simulink model "Ex_3"  (R2023b)
settings: Solver=VariableStepAuto  StartTime=0.0  StopTime=10.0  RelTol=1e-3
undefined symbols (not defined in the file): X, Y, Z
libraries: nesl_utility x21, sm_lib x20, robotcorelib x2, simulink x2
settings Model: Creator=aless  LastModifiedBy=aless

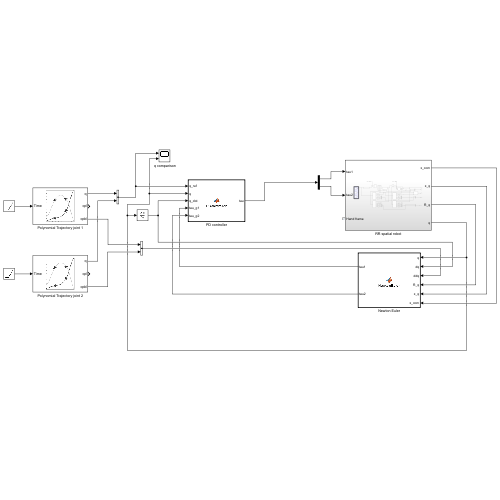
[thumbnail: Simulink's stored preview of the top-level diagram]
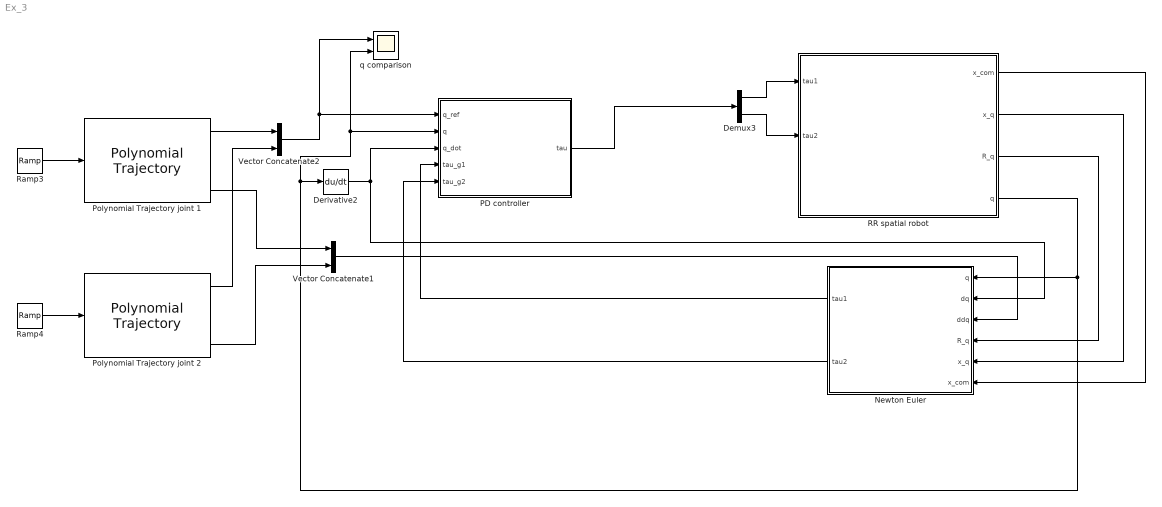
== system Ex_3 ==
  " q comparison" : Scope  NumInputPorts=2
  Demux3 : Demux  Outputs=2
  Derivative2 : Derivative
  Newton Euler : MATLAB Function  TreatAsAtomicUnit=on
  PD controller : MATLAB Function  TreatAsAtomicUnit=on
  Polynomial Trajectory joint 1 : robotcorelib/Polynomial Trajectory  WaypointSource=Internal  Waypoints=[ deg2rad(-25), deg2rad(100)]  TimePoints=[ 0, 10]  TimeInterval=[ 1, 4 ]  Method=Cubic Polynomial  ParameterSource=Internal  VelocityBoundaryCondition=zeros( 1, 2 )  AccelerationBoundaryCondition=zeros( 2, 5 )  SimulateUsing=Interpreted execution
  Polynomial Trajectory joint 2 : robotcorelib/Polynomial Trajectory  WaypointSource=Internal  Waypoints=[ deg2rad(45), deg2rad(80)]  TimePoints=[ 0, 10]  TimeInterval=[ 1, 4 ]  Method=Cubic Polynomial  ParameterSource=Internal  VelocityBoundaryCondition=zeros( 1, 2 )  AccelerationBoundaryCondition=zeros( 2, 5 )  SimulateUsing=Interpreted execution
  RR spatial robot : Subsystem
  Ramp3 : simulink/Sources/Ramp  slope=1  start=0  InitialOutput=0
  Ramp4 : simulink/Sources/Ramp  slope=1  start=0  InitialOutput=0
  Vector Concatenate1 : Concatenate
  Vector Concatenate2 : Concatenate
  wires:
  Demux3/2 -> RR spatial robot/2(tau2)
  Polynomial Trajectory joint 1/1 -> Vector Concatenate2/1
  Polynomial Trajectory joint 2/1 -> Vector Concatenate2/2
  Vector Concatenate1/1 -> Newton Euler/3(ddq)
  Polynomial Trajectory joint 1/3 -> Vector Concatenate1/1
  Newton Euler/2(tau2) -> PD controller/5(tau_g2)
  PD controller/1(tau) -> Demux3/1
  Polynomial Trajectory joint 2/3 -> Vector Concatenate1/2
  RR spatial robot/3(R_q) -> Newton Euler/4(R_q)
  Newton Euler/1(tau1) -> PD controller/4(tau_g1)
  RR spatial robot/4(q) -> Derivative2/1, " q comparison"/2, PD controller/2(q), Newton Euler/1(q)
  Ramp4/1 -> Polynomial Trajectory joint 2/1
  Ramp3/1 -> Polynomial Trajectory joint 1/1
  Derivative2/1 -> Newton Euler/2(dq), PD controller/3(q_dot)
  Demux3/1 -> RR spatial robot/1(tau1)
  Vector Concatenate2/1 -> " q comparison"/1, PD controller/1(q_ref)
  RR spatial robot/1(x_com) -> Newton Euler/6(x_com)
  RR spatial robot/2(x_q) -> Newton Euler/5(x_q)

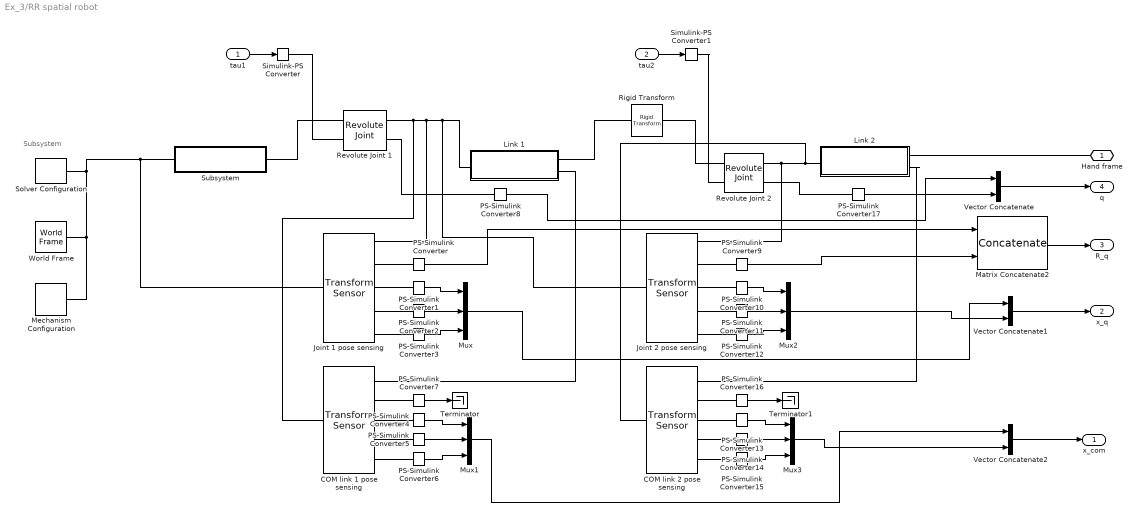
== system Ex_3/RR spatial robot ==
  note: Subsystem
  tau1 : Inport
  tau2 : Inport  Port=2
  COM link 1 pose sensing : sm_lib/Frames and Transforms/Transform Sensor  MeasurementFrame=Base  RotationSequence=XYX  SenseAngle=off  SenseAxis=off  SenseQ=off  SenseR=on  SenseRotationSequence=off  SenseOmegaX=off  SenseOmegaY=off  SenseOmegaZ=off  SenseOmega=off  SenseQDot=off  SenseRDot=off  SenseRotationSequenceDot=off  SenseAlphaX=off  SenseAlphaY=off  SenseAlphaZ=off  SenseAlpha=off  SenseQDDot=off  SenseRDDot=off  SenseX=on  SenseY=on  SenseZ=on  SenseXYZ=off  SenseRad=off  SenseAzim=off  SenseDist=off  SenseInc=off  SenseXDot=off  SenseYDot=off  SenseZDot=off  SenseXYZDot=off  SenseRadDot=off  SenseAzimDot=off  SenseDistDot=off  SenseIncDot=off  SenseXDDot=off  SenseYDDot=off  SenseZDDot=off  SenseXYZDDot=off  SenseRadDDot=off  SenseAzimDDot=off  SenseDistDDot=off  SenseIncDDot=off
  COM link 2 pose sensing : sm_lib/Frames and Transforms/Transform Sensor  MeasurementFrame=Base  RotationSequence=XYX  SenseAngle=off  SenseAxis=off  SenseQ=off  SenseR=on  SenseRotationSequence=off  SenseOmegaX=off  SenseOmegaY=off  SenseOmegaZ=off  SenseOmega=off  SenseQDot=off  SenseRDot=off  SenseRotationSequenceDot=off  SenseAlphaX=off  SenseAlphaY=off  SenseAlphaZ=off  SenseAlpha=off  SenseQDDot=off  SenseRDDot=off  SenseX=on  SenseY=on  SenseZ=on  SenseXYZ=off  SenseRad=off  SenseAzim=off  SenseDist=off  SenseInc=off  SenseXDot=off  SenseYDot=off  SenseZDot=off  SenseXYZDot=off  SenseRadDot=off  SenseAzimDot=off  SenseDistDot=off  SenseIncDot=off  SenseXDDot=off  SenseYDDot=off  SenseZDDot=off  SenseXYZDDot=off  SenseRadDDot=off  SenseAzimDDot=off  SenseDistDDot=off  SenseIncDDot=off
  Joint 1 pose sensing : sm_lib/Frames and Transforms/Transform Sensor  MeasurementFrame=Base  RotationSequence=XYX  SenseAngle=off  SenseAxis=off  SenseQ=off  SenseR=on  SenseRotationSequence=off  SenseOmegaX=off  SenseOmegaY=off  SenseOmegaZ=off  SenseOmega=off  SenseQDot=off  SenseRDot=off  SenseRotationSequenceDot=off  SenseAlphaX=off  SenseAlphaY=off  SenseAlphaZ=off  SenseAlpha=off  SenseQDDot=off  SenseRDDot=off  SenseX=on  SenseY=on  SenseZ=on  SenseXYZ=off  SenseRad=off  SenseAzim=off  SenseDist=off  SenseInc=off  SenseXDot=off  SenseYDot=off  SenseZDot=off  SenseXYZDot=off  SenseRadDot=off  SenseAzimDot=off  SenseDistDot=off  SenseIncDot=off  SenseXDDot=off  SenseYDDot=off  SenseZDDot=off  SenseXYZDDot=off  SenseRadDDot=off  SenseAzimDDot=off  SenseDistDDot=off  SenseIncDDot=off
  Joint 2 pose sensing : sm_lib/Frames and Transforms/Transform Sensor  MeasurementFrame=Base  RotationSequence=XYX  SenseAngle=off  SenseAxis=off  SenseQ=off  SenseR=on  SenseRotationSequence=off  SenseOmegaX=off  SenseOmegaY=off  SenseOmegaZ=off  SenseOmega=off  SenseQDot=off  SenseRDot=off  SenseRotationSequenceDot=off  SenseAlphaX=off  SenseAlphaY=off  SenseAlphaZ=off  SenseAlpha=off  SenseQDDot=off  SenseRDDot=off  SenseX=on  SenseY=on  SenseZ=on  SenseXYZ=off  SenseRad=off  SenseAzim=off  SenseDist=off  SenseInc=off  SenseXDot=off  SenseYDot=off  SenseZDot=off  SenseXYZDot=off  SenseRadDot=off  SenseAzimDot=off  SenseDistDot=off  SenseIncDot=off  SenseXDDot=off  SenseYDDot=off  SenseZDDot=off  SenseXYZDDot=off  SenseRadDDot=off  SenseAzimDDot=off  SenseDistDDot=off  SenseIncDDot=off
  Link 1 : Subsystem
  Link 2 : Subsystem
  Matrix Concatenate2 : Concatenate  Mode=Multidimensional array  ConcatenateDimension=3
  Mechanism Configuration : sm_lib/Utilities/Mechanism Configuration  UniformGravity=Constant  GravityVector=[0 0 -9.80665]  GravityVectorUnits=m/s^2  LinearizationDelta=0.001  JointModeTransitionNonlinearIterations=2
  Mux{,1..3} (4 alike) : Mux  Inputs=3
  PS-Simulink Converter{,1..17} (18 alike) : nesl_utility/PS-Simulink Converter  PhysicalDomain=network_engine_domain  SubClassName=ps_output  LeftPortType=input  RightPortType=output  PseudoPeriodic=off  Frequencies=[]  VectorFormat=inherit  Unit=inherit  AffineConversion=off
  Revolute Joint 1 : sm_lib/Joints/Revolute Joint  JointMode=Normal  SenseConstraintForce=off  SenseConstraintForceX=off  SenseConstraintForceY=off  SenseConstraintForceZ=off  SenseConstraintTorque=off  SenseConstraintTorqueX=off  SenseConstraintTorqueY=off  SenseConstraintTorqueZ=off  SenseTotalForce=off  SenseTotalForceX=off  SenseTotalForceY=off  SenseTotalForceZ=off  SenseTotalTorque=off  SenseTotalTorqueX=off  SenseTotalTorqueY=off  SenseTotalTorqueZ=off  CompositeWrenchDir=FollowerOnBase  CompositeWrenchFrame=BaseFrame  EquilibriumPosition=0  EquilibriumPositionUnits=deg  SpringStiffness=0  SpringStiffnessUnits=N*m/deg  DampingCoefficient=0  DampingCoefficientUnits=N*m*s/rad  TorqueActuationMode=InputTorque  MotionActuationMode=ComputedMotion  SensePosition=on  SenseVelocity=off  SenseAcceleration=off  SenseTorqueForce=off  SenseLowerLimitTorqueForce=off  SenseUpperLimitTorqueForce=off  LowerLimitSpecify=off  LowerLimitBound=-90  LowerLimitBoundUnits=deg  LowerLimitStiffness=1e4  LowerLimitStiffnessUnits=N*m/deg  LowerLimitDamping=10  LowerLimitDampingUnits=N*m/(deg/s)  LowerLimitTransitionRegionWidth=0.1  LowerLimitTransitionRegionWidthUnits=deg  UpperLimitSpecify=off  UpperLimitBound=90  UpperLimitBoundUnits=deg  UpperLimitStiffness=1e4  UpperLimitStiffnessUnits=N*m/deg  UpperLimitDamping=10  UpperLimitDampingUnits=N*m/(deg/s)  UpperLimitTransitionRegionWidth=0.1  UpperLimitTransitionRegionWidthUnits=deg  PositionTargetSpecify=on  PositionTargetPriority=High  PositionTargetValue=-25  PositionTargetValueUnits=deg  VelocityTargetSpecify=off  VelocityTargetPriority=High  VelocityTargetValue=0  VelocityTargetValueUnits=deg/s
  Revolute Joint 2 : sm_lib/Joints/Revolute Joint  JointMode=Normal  SenseConstraintForce=off  SenseConstraintForceX=off  SenseConstraintForceY=off  SenseConstraintForceZ=off  SenseConstraintTorque=off  SenseConstraintTorqueX=off  SenseConstraintTorqueY=off  SenseConstraintTorqueZ=off  SenseTotalForce=off  SenseTotalForceX=off  SenseTotalForceY=off  SenseTotalForceZ=off  SenseTotalTorque=off  SenseTotalTorqueX=off  SenseTotalTorqueY=off  SenseTotalTorqueZ=off  CompositeWrenchDir=FollowerOnBase  CompositeWrenchFrame=BaseFrame  EquilibriumPosition=0  EquilibriumPositionUnits=deg  SpringStiffness=0  SpringStiffnessUnits=N*m/deg  DampingCoefficient=0  DampingCoefficientUnits=N*m*s/rad  TorqueActuationMode=InputTorque  MotionActuationMode=ComputedMotion  SensePosition=on  SenseVelocity=off  SenseAcceleration=off  SenseTorqueForce=off  SenseLowerLimitTorqueForce=off  SenseUpperLimitTorqueForce=off  LowerLimitSpecify=off  LowerLimitBound=-90  LowerLimitBoundUnits=deg  LowerLimitStiffness=1e4  LowerLimitStiffnessUnits=N*m/deg  LowerLimitDamping=10  LowerLimitDampingUnits=N*m/(deg/s)  LowerLimitTransitionRegionWidth=0.1  LowerLimitTransitionRegionWidthUnits=deg  UpperLimitSpecify=off  UpperLimitBound=90  UpperLimitBoundUnits=deg  UpperLimitStiffness=1e4  UpperLimitStiffnessUnits=N*m/deg  UpperLimitDamping=10  UpperLimitDampingUnits=N*m/(deg/s)  UpperLimitTransitionRegionWidth=0.1  UpperLimitTransitionRegionWidthUnits=deg  PositionTargetSpecify=on  PositionTargetPriority=High  PositionTargetValue=45  PositionTargetValueUnits=deg  VelocityTargetSpecify=off  VelocityTargetPriority=High  VelocityTargetValue=0  VelocityTargetValueUnits=deg/s
  Rigid Transform : sm_lib/Frames and Transforms/Rigid Transform  TranslationMethod=None  TranslationStandardOffset=0  TranslationStandardOffsetUnits=m  TranslationStandardAxis=+Z  TranslationCartesianOffset=[0 0 0]  TranslationCartesianOffsetUnits=m  TranslationROffset=0  TranslationROffsetUnits=m  TranslationZOffset=0  TranslationZOffsetUnits=m  TranslationThetaOffset=0  TranslationThetaOffsetUnits=deg  RotationMethod=StandardAxis  RotationAngleUnits=deg  RotationStandardAxis=+Y  RotationAngle=90  RotationArbitraryAxis=[0 0 1]  FollAlignAxisA=+X  BaseAlignAxisA=+Y  FollAlignAxisB=+Y  BaseAlignAxisB=+Z  RotationSequenceAxes=FollowerAxes  RotationSequence=XYX  RotationSequenceAngles=[0 0 0]  RotationSequenceAnglesUnits=deg  RotationMatrix=[1 0 0; 0 1 0; 0 0 1]  Quaternion=[1 0 0 0]
  Simulink-PS Converter : nesl_utility/Simulink-PS Converter  PhysicalDomain=network_engine_domain  SubClassName=ps_input  LeftPortType=input  RightPortType=output  PseudoPeriodic=off  Frequencies=[]  NoiseDistribution=none  NoiseParameters=[]  Unit=1  AffineConversion=off  FilteringAndDerivatives=provide  SimscapeFilterOrder=1  InputFilterTimeConstant=0.001  UdotUserProvided=0
  Simulink-PS Converter1 : nesl_utility/Simulink-PS Converter  PhysicalDomain=network_engine_domain  SubClassName=ps_input  LeftPortType=input  RightPortType=output  PseudoPeriodic=off  Frequencies=[]  NoiseDistribution=none  NoiseParameters=[]  Unit=1  AffineConversion=off  FilteringAndDerivatives=provide  SimscapeFilterOrder=1  InputFilterTimeConstant=0.001  UdotUserProvided=0
  Solver Configuration : nesl_utility/Solver Configuration  PhysicalDomain=network_engine_domain  SubClassName=solver  LeftPortType=input  RightPortType=generic  Tones=[]  Harmonics=[]  SimulateNoise=off  Profile=off  UseLocalSampling=off  EnableSwitchedLinearOptims=on  FrequencyDomain=off  UseCCode=off  RelTol=0.001  AbsTol=1e-06  MinStep=1e-09  ToWorkspace=off  RevertToSquareIcSolve=off  NumHomotopyIterations=100  PhasorMode=off  PhasorModeNumHarmonics=1  ConsistencySolver=NEWTON_XTOL_AFTER_FTOL  IndexReductionMethod=DerivativeReplacement  DoDC=off  ResidualTolerance=1e-09  ConsistencyTolSource=GLOBAL  ConsistencyAbsTol=0.001  ConsistencyRelTol=0.001  ConsistencyTolFactor=0.001  UseLocalSolver=off  LocalSolverChoice=NE_BACKWARD_EULER_ADVANCER  ResolveIndetEquations=on  FunctionEvalNumThread=1  LocalSolverSampleTime=0.001  DoFixedCost=off  MaxNonlinIter=3  MaxModeIter=2  ComputeImpulses=off  ImpulseIterations=2  LinearAlgebra=Sparse  LinearAlgebraNumThread=0  EquationFormulation=NE_TIME_EF  DelaysMemoryBudget=1024  AutomaticFiltering=on  FilteringTimeConstant=0.001  PartitionStorageMethod=AS_NEEDED  PartitionMemoryBudget=1024  PartitionMethod=FAST  MultibodyUseLocalSolver=off  MultibodyLocalSolverChoice=ODE1  MultibodyLocalSolverSampleTime=0.001
  Subsystem : Subsystem
  Terminator : Terminator
  Terminator1 : Terminator
  Vector Concatenate : Concatenate  Mode=Multidimensional array  ConcatenateDimension=2
  Vector Concatenate1 : Concatenate  Mode=Multidimensional array  ConcatenateDimension=2
  Vector Concatenate2 : Concatenate  Mode=Multidimensional array  ConcatenateDimension=2
  World Frame : sm_lib/Frames and Transforms/World Frame
  Hand frame : PMIOPort  Side=Left
  x_com : Outport
  x_q : Outport  Port=2
  R_q : Outport  Port=3
  q : Outport  Port=4
  wires:
  PS-Simulink Converter4/1 -> Mux1/1
  Vector Concatenate2/1 -> x_com/1
  PS-Simulink Converter7/1 -> Terminator/1
  Mux2/1 -> Vector Concatenate1/2
  tau1/1 -> Simulink-PS Converter/1
  PS-Simulink Converter2/1 -> Mux/2
  PS-Simulink Converter13/1 -> Mux3/1
  PS-Simulink Converter1/1 -> Mux/1
  Mux1/1 -> Vector Concatenate2/1
  PS-Simulink Converter16/1 -> Terminator1/1
  Vector Concatenate1/1 -> x_q/1
  PS-Simulink Converter6/1 -> Mux1/3
  PS-Simulink Converter12/1 -> Mux2/3
  PS-Simulink Converter9/1 -> Matrix Concatenate2/2
  PS-Simulink Converter8/1 -> Vector Concatenate/1
  Vector Concatenate/1 -> q/1
  Matrix Concatenate2/1 -> R_q/1
  PS-Simulink Converter5/1 -> Mux1/2
  PS-Simulink Converter3/1 -> Mux/3
  PS-Simulink Converter11/1 -> Mux2/2
  PS-Simulink Converter14/1 -> Mux3/2
  PS-Simulink Converter/1 -> Matrix Concatenate2/1
  PS-Simulink Converter15/1 -> Mux3/3
  Mux/1 -> Vector Concatenate1/1
  tau2/1 -> Simulink-PS Converter1/1
  PS-Simulink Converter10/1 -> Mux2/1
  PS-Simulink Converter17/1 -> Vector Concatenate/2
  Mux3/1 -> Vector Concatenate2/2
  connections:
  Link 2/RConn1 -- Joint 2 pose sensing/RConn1 -- Revolute Joint 2/RConn1 -- COM link 2 pose sensing/LConn1
  Revolute Joint 1/RConn1 -- COM link 1 pose sensing/LConn1 -- Joint 2 pose sensing/LConn1 -- Link 1/RConn1 -- Joint 1 pose sensing/RConn1
  World Frame/RConn1 -- Joint 1 pose sensing/LConn1 -- Subsystem/LConn1 -- Solver Configuration/RConn1 -- Mechanism Configuration/RConn1
  COM link 1 pose sensing/RConn4 -- PS-Simulink Converter5/LConn1
  Link 1/LConn1 -- Rigid Transform/LConn1
  PS-Simulink Converter1/LConn1 -- Joint 1 pose sensing/RConn3
  Joint 2 pose sensing/RConn5 -- PS-Simulink Converter12/LConn1
  Link 2/LConn2 -- COM link 2 pose sensing/RConn1
  COM link 1 pose sensing/RConn3 -- PS-Simulink Converter4/LConn1
  COM link 2 pose sensing/RConn2 -- PS-Simulink Converter16/LConn1
  Joint 2 pose sensing/RConn4 -- PS-Simulink Converter11/LConn1
  Joint 2 pose sensing/RConn2 -- PS-Simulink Converter9/LConn1
  COM link 2 pose sensing/RConn5 -- PS-Simulink Converter15/LConn1
  PS-Simulink Converter17/LConn1 -- Revolute Joint 2/RConn2
  Simulink-PS Converter1/RConn1 -- Revolute Joint 2/LConn2
  COM link 1 pose sensing/RConn2 -- PS-Simulink Converter7/LConn1
  Joint 1 pose sensing/RConn4 -- PS-Simulink Converter2/LConn1
  Simulink-PS Converter/RConn1 -- Revolute Joint 1/LConn2
  Revolute Joint 1/LConn1 -- Subsystem/RConn1
  Joint 1 pose sensing/RConn5 -- PS-Simulink Converter3/LConn1
  Link 1/LConn2 -- COM link 1 pose sensing/RConn1
  Link 2/LConn1 -- Hand frame/RConn1
  COM link 1 pose sensing/RConn5 -- PS-Simulink Converter6/LConn1
  PS-Simulink Converter10/LConn1 -- Joint 2 pose sensing/RConn3
  Rigid Transform/RConn1 -- Revolute Joint 2/LConn1
  Revolute Joint 1/RConn2 -- PS-Simulink Converter8/LConn1
  COM link 2 pose sensing/RConn3 -- PS-Simulink Converter13/LConn1
  COM link 2 pose sensing/RConn4 -- PS-Simulink Converter14/LConn1
  Joint 1 pose sensing/RConn2 -- PS-Simulink Converter/LConn1

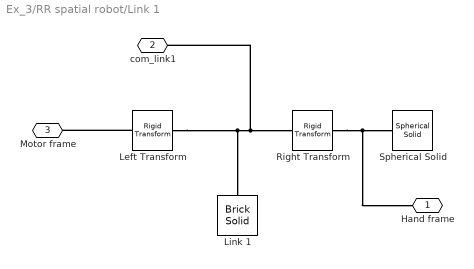
== system Ex_3/RR spatial robot/Link 1 ==
  Left Transform : sm_lib/Frames and Transforms/Rigid Transform  TranslationMethod=StandardAxis  TranslationStandardOffset=20  TranslationStandardOffsetUnits=cm  TranslationStandardAxis=+X  TranslationCartesianOffset=[0 0 0]  TranslationCartesianOffsetUnits=m  TranslationROffset=0  TranslationROffsetUnits=m  TranslationZOffset=0  TranslationZOffsetUnits=m  TranslationThetaOffset=0  TranslationThetaOffsetUnits=deg  RotationMethod=None  RotationAngleUnits=deg  RotationStandardAxis=+Z  RotationAngle=0.0  RotationArbitraryAxis=[0 0 1]  FollAlignAxisA=+X  BaseAlignAxisA=+Y  FollAlignAxisB=+Y  BaseAlignAxisB=+Z  RotationSequenceAxes=FollowerAxes  RotationSequence=XYX  RotationSequenceAngles=[0 0 0]  RotationSequenceAnglesUnits=deg  RotationMatrix=[1 0 0; 0 1 0; 0 0 1]  Quaternion=[1 0 0 0]
  Link 1 : sm_lib/Body Elements/Brick Solid  GraphicAmbientColor=[0.15 0.15 0.15 1.0]  BasedOnType=Mass  BrickDimensions=[0.4 0.01 0.01]  BrickDimensionsUnits=m  CenterOfMass=[0 0 0]  CenterOfMassUnits=m  GraphicDiffuseColor=[1.0 0.0 0.2]  Density=1000  DensityUnits=kg/m^3  DoExposeReferenceFrame=on  GraphicEmissiveColor=[0.0 0.0 0.0 1.0]  ExportEntireGeometry=off  SerializedFrames=<Frames/>  MarkerShape=Sphere  MarkerSize=10  GraphicType=FromGeometry  InertiaType=CalculateFromGeometry  Mass=2  MassUnits=kg  MomentsOfInertia=[1 1 1]  MomentsOfInertiaUnits=kg*m^2  GraphicOpacity=1.0  ProductsOfInertia=[0 0 0]  ProductsOfInertiaUnits=kg*m^2  GraphicShininess=75  GraphicSpecularColor=[0.5 0.5 0.5 1.0]  GraphicVisPropType=SimpleVisualProperties
  Right Transform : sm_lib/Frames and Transforms/Rigid Transform  TranslationMethod=StandardAxis  TranslationStandardOffset=20  TranslationStandardOffsetUnits=cm  TranslationStandardAxis=+X  TranslationCartesianOffset=[0 0 0]  TranslationCartesianOffsetUnits=m  TranslationROffset=0  TranslationROffsetUnits=m  TranslationZOffset=0  TranslationZOffsetUnits=m  TranslationThetaOffset=0  TranslationThetaOffsetUnits=deg  RotationMethod=None  RotationAngleUnits=deg  RotationStandardAxis=+Y  RotationAngle=90  RotationArbitraryAxis=[0 0 1]  FollAlignAxisA=+X  BaseAlignAxisA=+Y  FollAlignAxisB=+Y  BaseAlignAxisB=+Z  RotationSequenceAxes=FollowerAxes  RotationSequence=XYX  RotationSequenceAngles=[0 0 0]  RotationSequenceAnglesUnits=deg  RotationMatrix=[1 0 0; 0 1 0; 0 0 1]  Quaternion=[1 0 0 0]
  Spherical Solid : sm_lib/Body Elements/Spherical Solid  GraphicAmbientColor=[0.15 0.15 0.15 1.0]  BasedOnType=Mass  CenterOfMass=[0 0 0]  CenterOfMassUnits=m  GraphicDiffuseColor=[0.2 0.4 1.0]  Density=1000  DensityUnits=kg/m^3  DoExposeReferenceFrame=on  GraphicEmissiveColor=[0.0 0.0 0.0 1.0]  ExportEntireGeometry=off  SerializedExposedGeometries=<exposedGeometries/>  SerializedFrames=<Frames/>  MarkerShape=Sphere  MarkerSize=10  GraphicType=FromGeometry  InertiaType=CalculateFromGeometry  Mass=0  MassUnits=kg  MomentsOfInertia=[1 1 1]  MomentsOfInertiaUnits=kg*m^2  GraphicOpacity=1.0  ProductsOfInertia=[0 0 0]  ProductsOfInertiaUnits=kg*m^2  GraphicShininess=75  GraphicSpecularColor=[0.5 0.5 0.5 1.0]  SphereRadius=2  SphereRadiusUnits=cm  GraphicVisPropType=SimpleVisualProperties
  Hand frame : PMIOPort  Side=Left
  com_link1 : PMIOPort  Port=2  Side=Left
  Motor frame : PMIOPort  Port=3  Side=Right
  connections:
  Left Transform/RConn1 -- com_link1/RConn1 -- Right Transform/LConn1 -- Link 1/RConn1
  Left Transform/LConn1 -- Motor frame/RConn1
  Right Transform/RConn1 -- Hand frame/RConn1 -- Spherical Solid/RConn1

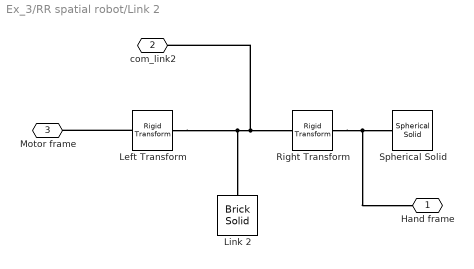
== system Ex_3/RR spatial robot/Link 2 ==
  Left Transform : sm_lib/Frames and Transforms/Rigid Transform  TranslationMethod=StandardAxis  TranslationStandardOffset=15  TranslationStandardOffsetUnits=cm  TranslationStandardAxis=+X  TranslationCartesianOffset=[0 0 0]  TranslationCartesianOffsetUnits=m  TranslationROffset=0  TranslationROffsetUnits=m  TranslationZOffset=0  TranslationZOffsetUnits=m  TranslationThetaOffset=0  TranslationThetaOffsetUnits=deg  RotationMethod=None  RotationAngleUnits=deg  RotationStandardAxis=+Z  RotationAngle=0.0  RotationArbitraryAxis=[0 0 1]  FollAlignAxisA=+X  BaseAlignAxisA=+Y  FollAlignAxisB=+Y  BaseAlignAxisB=+Z  RotationSequenceAxes=FollowerAxes  RotationSequence=XYX  RotationSequenceAngles=[0 0 0]  RotationSequenceAnglesUnits=deg  RotationMatrix=[1 0 0; 0 1 0; 0 0 1]  Quaternion=[1 0 0 0]
  Link 2 : sm_lib/Body Elements/Brick Solid  GraphicAmbientColor=[0.15 0.15 0.15 1.0]  BasedOnType=Mass  BrickDimensions=[0.3 0.01 0.01]  BrickDimensionsUnits=m  CenterOfMass=[0 0 0]  CenterOfMassUnits=m  GraphicDiffuseColor=[1.0 0.0 0.2]  Density=1000  DensityUnits=kg/m^3  DoExposeReferenceFrame=on  GraphicEmissiveColor=[0.0 0.0 0.0 1.0]  ExportEntireGeometry=off  SerializedFrames=<Frames/>  MarkerShape=Sphere  MarkerSize=10  GraphicType=FromGeometry  InertiaType=CalculateFromGeometry  Mass=6.5  MassUnits=kg  MomentsOfInertia=[1 1 1]  MomentsOfInertiaUnits=kg*m^2  GraphicOpacity=1.0  ProductsOfInertia=[0 0 0]  ProductsOfInertiaUnits=kg*m^2  GraphicShininess=75  GraphicSpecularColor=[0.5 0.5 0.5 1.0]  GraphicVisPropType=SimpleVisualProperties
  Right Transform : sm_lib/Frames and Transforms/Rigid Transform  TranslationMethod=StandardAxis  TranslationStandardOffset=15  TranslationStandardOffsetUnits=cm  TranslationStandardAxis=+X  TranslationCartesianOffset=[0 0 0]  TranslationCartesianOffsetUnits=m  TranslationROffset=0  TranslationROffsetUnits=m  TranslationZOffset=0  TranslationZOffsetUnits=m  TranslationThetaOffset=0  TranslationThetaOffsetUnits=deg  RotationMethod=None  RotationAngleUnits=deg  RotationStandardAxis=+Z  RotationAngle=0.0  RotationArbitraryAxis=[0 0 1]  FollAlignAxisA=+X  BaseAlignAxisA=+Y  FollAlignAxisB=+Y  BaseAlignAxisB=+Z  RotationSequenceAxes=FollowerAxes  RotationSequence=XYX  RotationSequenceAngles=[0 0 0]  RotationSequenceAnglesUnits=deg  RotationMatrix=[1 0 0; 0 1 0; 0 0 1]  Quaternion=[1 0 0 0]
  Spherical Solid : sm_lib/Body Elements/Spherical Solid  GraphicAmbientColor=[0.15 0.15 0.15 1.0]  BasedOnType=Mass  CenterOfMass=[0 0 0]  CenterOfMassUnits=m  GraphicDiffuseColor=[0.2 0.4 1.0]  Density=1000  DensityUnits=kg/m^3  DoExposeReferenceFrame=on  GraphicEmissiveColor=[0.0 0.0 0.0 1.0]  ExportEntireGeometry=off  SerializedExposedGeometries=<exposedGeometries/>  SerializedFrames=<Frames/>  MarkerShape=Sphere  MarkerSize=10  GraphicType=FromGeometry  InertiaType=CalculateFromGeometry  Mass=0  MassUnits=kg  MomentsOfInertia=[1 1 1]  MomentsOfInertiaUnits=kg*m^2  GraphicOpacity=1.0  ProductsOfInertia=[0 0 0]  ProductsOfInertiaUnits=kg*m^2  GraphicShininess=75  GraphicSpecularColor=[0.5 0.5 0.5 1.0]  SphereRadius=2  SphereRadiusUnits=cm  GraphicVisPropType=SimpleVisualProperties
  Hand frame : PMIOPort  Side=Left
  com_link2 : PMIOPort  Port=2  Side=Left
  Motor frame : PMIOPort  Port=3  Side=Right
  connections:
  com_link2/RConn1 -- Right Transform/LConn1 -- Left Transform/RConn1 -- Link 2/RConn1
  Left Transform/LConn1 -- Motor frame/RConn1
  Right Transform/RConn1 -- Hand frame/RConn1 -- Spherical Solid/RConn1

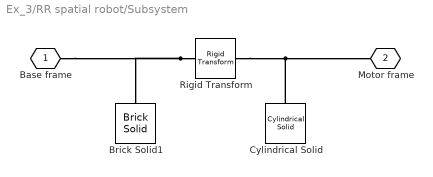
== system Ex_3/RR spatial robot/Subsystem ==
  Brick Solid1 : sm_lib/Body Elements/Brick Solid  GraphicAmbientColor=[0.15 0.15 0.15 1.0]  BasedOnType=Density  BrickDimensions=[30 30 5]  BrickDimensionsUnits=cm  CenterOfMass=[0 0 0]  CenterOfMassUnits=m  GraphicDiffuseColor=[0.5 0.5 0.5]  Density=1000  DensityUnits=kg/m^3  DoExposeReferenceFrame=on  GraphicEmissiveColor=[0.0 0.0 0.0 1.0]  ExportEntireGeometry=off  SerializedFrames=<Frames/>  MarkerShape=Sphere  MarkerSize=10  GraphicType=FromGeometry  InertiaType=CalculateFromGeometry  Mass=1  MassUnits=kg  MomentsOfInertia=[1 1 1]  MomentsOfInertiaUnits=kg*m^2  GraphicOpacity=1.0  ProductsOfInertia=[0 0 0]  ProductsOfInertiaUnits=kg*m^2  GraphicShininess=75  GraphicSpecularColor=[0.5 0.5 0.5 1.0]  GraphicVisPropType=SimpleVisualProperties
  Cylindrical Solid : sm_lib/Body Elements/Cylindrical Solid  GraphicAmbientColor=[0.15 0.15 0.15 1.0]  BasedOnType=Density  CenterOfMass=[0 0 0]  CenterOfMassUnits=m  GraphicDiffuseColor=[0.2 0.2 0.2]  CylinderLength=5  CylinderLengthUnits=cm  CylinderRadius=3  CylinderRadiusUnits=cm  Density=1000  DensityUnits=kg/m^3  DoExposeReferenceFrame=on  GraphicEmissiveColor=[0.0 0.0 0.0 1.0]  ExportEntireGeometry=off  SerializedFrames=<Frames/>  MarkerShape=Sphere  MarkerSize=10  GraphicType=FromGeometry  InertiaType=CalculateFromGeometry  Mass=1  MassUnits=kg  MomentsOfInertia=[1 1 1]  MomentsOfInertiaUnits=kg*m^2  GraphicOpacity=1.0  ProductsOfInertia=[0 0 0]  ProductsOfInertiaUnits=kg*m^2  GraphicShininess=75  GraphicSpecularColor=[0.5 0.5 0.5 1.0]  GraphicVisPropType=SimpleVisualProperties
  Rigid Transform : sm_lib/Frames and Transforms/Rigid Transform  TranslationMethod=StandardAxis  TranslationStandardOffset=5  TranslationStandardOffsetUnits=cm  TranslationStandardAxis=+Z  TranslationCartesianOffset=[0 0 0]  TranslationCartesianOffsetUnits=m  TranslationROffset=0  TranslationROffsetUnits=m  TranslationZOffset=0  TranslationZOffsetUnits=m  TranslationThetaOffset=0  TranslationThetaOffsetUnits=deg  RotationMethod=None  RotationAngleUnits=deg  RotationStandardAxis=+Z  RotationAngle=0.0  RotationArbitraryAxis=[0 0 1]  FollAlignAxisA=+X  BaseAlignAxisA=+Y  FollAlignAxisB=+Y  BaseAlignAxisB=+Z  RotationSequenceAxes=FollowerAxes  RotationSequence=XYX  RotationSequenceAngles=[0 0 0]  RotationSequenceAnglesUnits=deg  RotationMatrix=[1 0 0; 0 1 0; 0 0 1]  Quaternion=[1 0 0 0]
  Base frame : PMIOPort  Side=Left
  Motor frame : PMIOPort  Port=2  Side=Right
  connections:
  Rigid Transform/RConn1 -- Motor frame/RConn1 -- Cylindrical Solid/RConn1
  Rigid Transform/LConn1 -- Base frame/RConn1 -- Brick Solid1/RConn1

== matlab function Ex_3/PD controller ==
  data: q_ref input; tau output; q input; q_dot input; tau_g1 input; tau_g2 input
function tau  = PDcontroller(q_ref, q, q_dot, tau_g1, tau_g2)

Kp = 100;
Kd = 1;

tau = zeros(2,1);
tau(1) = Kp*(q_ref(1)-q(1))-Kd*q_dot(1)+tau_g1;
tau(2) = Kp*(q_ref(2)-q(2))-Kd*q_dot(2)+tau_g2;

end

== matlab function Ex_3/Newton Euler ==
  data: q input; tau1 output; dq input; ddq input; tau2 output; R_q input; x_q input; x_com input
function [tau1, tau2] = NewtonEuler(q, dq, ddq, R_q, x_q, x_com)
    % Function to compute joint torques using the Newton-Euler method
    % Inputs:
    %   q   - Joint positions
    %   dq  - Joint velocities
    %   ddq - Joint accelerations
    % Output:
    %   tau - Joint torques

    %% Forward Recursive Algorithm

    % Define the type and number of joints
    jointType = [0,0]; % 0 for revolute, 1 for prismatic
    jointNum = length(jointType); % Number of joints

    % Mass of the links
    m = [2; 6.5];

    % Length of the links (same for both links)
    l1 = 0.4;
    l2 = 0.3;

    % Calculate the moments of inertia for the first segment
    Ix1 = m(1)/12 * (l1^2);
    Iy1 = m(1)/12 * (l1^2);
    Iz1 = m(1)/12 * (l1^2);

    % Calculate the moments of inertia for the second segment
    Ix2 = m(2)/12 * (l2^2);
    Iy2 = m(2)/12 * (l2^2);
    Iz2 = m(2)/12 * (l2^2);

    % Inertia matrix for each segment
    Ic1 = diag([Ix1, Iy1, Iz1]);
    Ic2 = diag([Ix2, Iy2, Iz2]);

    % Gravitational acceleration vector
    g = [0; 0; 9.80665];

    % Unit vector along the z-axis
    Z = [0,0,1]';

    % Angular Velocity
    w = zeros(3,jointNum);
    w(:,1) = dq(1) * Z;
    w(:,2) = R_q(:,:,2)' * w(:,1) + dq(2) * Z;

    % Angular Acceleration
    w_dot = zeros(3,jointNum);
    w_dot(:,1) = ddq(1) * Z;
    w_dot(:,2) = R_q(:,:,2)' * w_dot(:,1) + cross(R_q(:,:,2)'*w(:,1),dq(2) * Z) + ddq(2) * Z;

    % Linear Acceleration
    v_dot = zeros(3,jointNum);
    v_dot(:,1) = R_q(:,:,1)' * g;
    v_dot(:,2) = R_q(:,:,2)' * (cross(w_dot(:,1),x_q(:,2)) + cross(w(:,1),cross(w(:,1),x_q(:,2))) + v_dot(:,1));

    % Linear Acceleration of COM
    v_dot_com = zeros(3,jointNum);
    v_dot_com(:,1) = cross(w_dot(:,1), x_com(:,1)) + cross(w(:,1),cross(w(:,1),x_com(:,1))) + v_dot(:,1);
    v_dot_com(:,2) = cross(w_dot(:,2), x_com(:,2)) + cross(w(:,2),cross(w(:,2),x_com(:,2))) + v_dot(:,2);

    % Force acting on COM
    F = zeros(3,jointNum);
    F(:,1) = m(1) * v_dot_com(:,1);
    F(:,2) = m(2) * v_dot_com(:,2);

    % Torque acting about COM
    N = zeros(3,jointNum);
    N(:,1) = Ic1 * w_dot(:,1) + cross(w(:,1), Ic1 * w(:,1));
    N(:,2) = Ic2 * w_dot(:,2) + cross(w(:,2), Ic2 * w(:,2));

    %% Backward Recursive Algorithm

    % Force acting on Joint
    f = zeros(3,jointNum);
    f(:,2) = F(:,2);
    f(:,1) = R_q(:,:,2) * f(:,2) + F(:,1);

    % Torque acting on Joint
    n = zeros(3,jointNum);
    n(:,2) = N(:,2) + cross(x_com(:,2), F(:,2));
    n(:,1) = N(:,1) + R_q(:,:,2) * n(:,2) + cross(x_com(:,1), F(:,1)) + cross(x_q(:,2), R_q(:,:,2) * f(:,2));

    % Torque acting on Join motion axis
    tau1 = n(:,1)' * Z;
    tau2 = n(:,2)' * Z;

end
